simulink model "p_regler_alleine"  (R2016b)
settings: Solver=FixedStepAuto  StartTime=0.0  StopTime=50.0  FixedStep=0.01  RelTol=1e-3
undefined symbols (not defined in the file or in its folder): K_TP, T_TP, transfunc
settings Model: Creator=Fritz  LastModifiedBy=Fritz

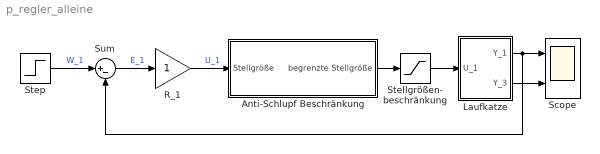
== system p_regler_alleine ==
  Anti-Schlupf Beschränkung : Subsystem
  Laufkatze : Subsystem
  R_1 : Gain
  Scope : Scope  NumInputPorts=2
  Stellgrößen- beschränkung : Saturate  UpperLimit=1  LowerLimit=-1
  Step : Step  Time=0  SampleTime=0
  Sum : Sum  Inputs=|+-
  wires:
  Step/1 -> Sum/1  "W_1"
  Anti-Schlupf Beschränkung/1(begrenzte Stellgröße) -> Stellgrößen- beschränkung/1
  Sum/1 -> R_1/1  "E_1"
  R_1/1 -> Anti-Schlupf Beschränkung/1(Stellgröße)  "U_1"
  Laufkatze/1(Y_1) -> Sum/2, Scope/1
  Stellgrößen- beschränkung/1 -> Laufkatze/1(U_1)
  Laufkatze/2(Y_3) -> Scope/2

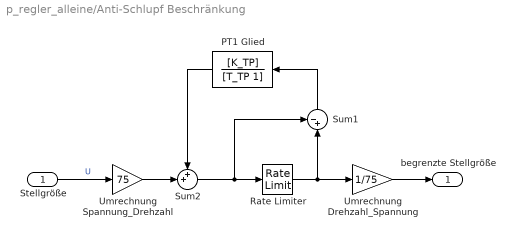
== system p_regler_alleine/Anti-Schlupf Beschränkung ==
  Stellgröße : Inport
  PT1 Glied : TransferFcn  Numerator=[K_TP]  Denominator=[T_TP 1]
  Rate Limiter : RateLimiter  RisingSlewLimit=9.57  FallingSlewLimit=-9.57  SampleTimeMode=inherited
  Sum1 : Sum  Inputs=-+|
  Sum2 : Sum  Inputs=++|
  Umrechnung Drehzahl_Spannung : Gain  Gain=1/75
  Umrechnung Spannung_Drehzahl : Gain  Gain=75
  begrenzte Stellgröße : Outport
  wires:
  Stellgröße/1 -> Umrechnung Spannung_Drehzahl/1  "U"
  Sum2/1 -> Sum1/1, Rate Limiter/1
  Sum1/1 -> PT1 Glied/1
  PT1 Glied/1 -> Sum2/1
  Rate Limiter/1 -> Umrechnung Drehzahl_Spannung/1, Sum1/2
  Umrechnung Spannung_Drehzahl/1 -> Sum2/2
  Umrechnung Drehzahl_Spannung/1 -> begrenzte Stellgröße/1

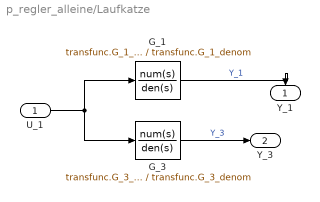
== system p_regler_alleine/Laufkatze ==
  U_1 : Inport
  G_1 : TransferFcn  Numerator=transfunc.G_1_numer  Denominator=transfunc.G_1_denom
  G_3 : TransferFcn  Numerator=transfunc.G_3_numer  Denominator=transfunc.G_3_denom
  Y_1 : Outport
  Y_3 : Outport  Port=2
  wires:
  U_1/1 -> G_3/1, G_1/1
  G_3/1 -> Y_3/1  "Y_3"
  G_1/1 -> Y_1/1  "Y_1"
